simulink model "sensor"  (R2014a)
settings: Solver=ode45  StartTime=0.0  StopTime=5  RelTol=1e-3
PreLoadFcn:
  | degconv=180/pi;
settings Model: Creator=RANGA  LastModifiedBy=RANGA
settings DataIOCC: LoadExternalInput=on

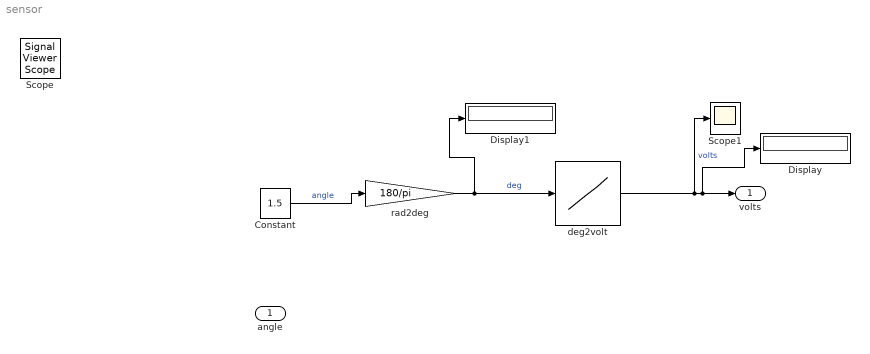
== system sensor ==
  angle : Inport
  Constant : Constant  Value=1.5
  Display : Display
  Display1 : Display
  Scope1 : Scope
      settings: ShowLegends=on
  deg2volt : Lookup_n-D  NumberOfTableDimensions=1  BreakpointsForDimension1=[0 90]  Table=[0.5 4.5]  ExtrapMethod=Clip  InternalRulePriority=Speed  RndMeth=Simplest  InputSameDT=on
  rad2deg : Gain  Gain=180/pi
  volts : Outport
  Scope : SignalViewerScope  IOType=viewer  NumInputPorts=2  ZoomMode=xonly  RefreshTime=0.035000
      settings: YMin=0~-5  YMax=5~5
  wires:
  deg2volt/1 -> Scope1/1, Display/1, volts/1  "volts"
  rad2deg/1 -> Display1/1, deg2volt/1  "deg"
  Constant/1 -> rad2deg/1  "angle"
